simulink model "model3"  (R2024b)
settings: Solver=VariableStepAuto  StartTime=0.0  StopTime=10  RelTol=1e-3
values from neighbouring files (symbols this model uses):
  A = [-3, 2; 1, -2]    [domaci3.m]
  B = [0; 2]    [domaci3.m]
  C = [0, 1]    [domaci3.m]
  K = acker(A, B, p_cl)    [domaci3.m]
  kr = 1 / dcgain(s * G0 / s)    [domaci3.m]
  L = acker(A', C', p_est)'    [domaci3.m]
  R = 5    [domaci3.m]
settings Model: Creator=neso  LastModifiedBy=neso

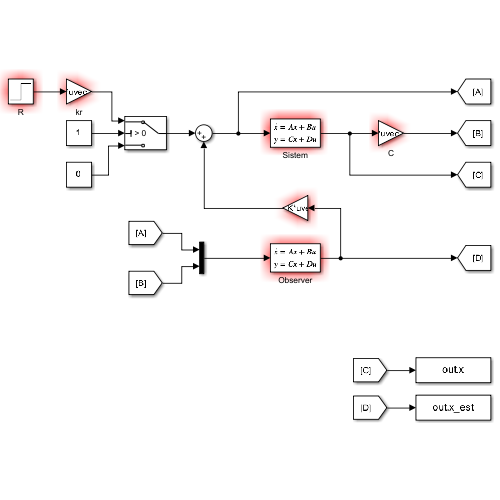
[thumbnail: Simulink's stored preview of the top-level diagram]
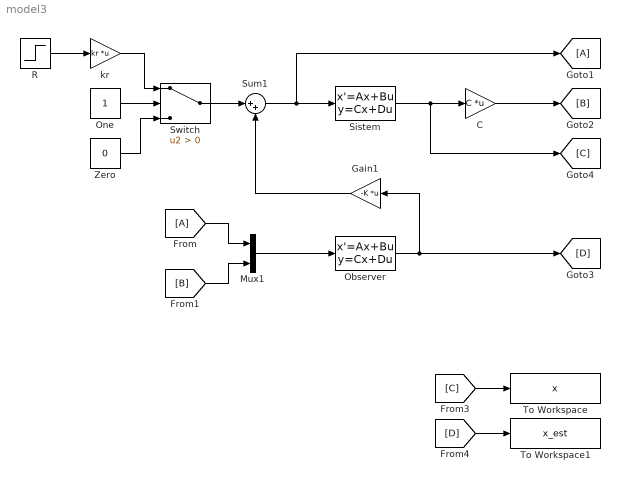
== system model3 ==
  C : Gain  Gain=C  Multiplication=Matrix(K*u) (u vector)
  From : From
  Gain1 : Gain  Gain=-K  Multiplication=Matrix(K*u) (u vector)
  Goto1 : Goto
  Mux1 : Mux  Inputs=2
  Observer : StateSpace  A=A - L .* C  B=[B, L]  C=[1, 0; 0, 1]  D=[0, 0; 0, 0]  InitialCondition=[0; 0]
  One : Constant  OutDataTypeStr=Inherit: Inherit via back propagation
  R : Step  Time=0  After=R  SampleTime=0
  Sistem : StateSpace  A=A  B=B  C=[1, 0; 0, 1]  D=[0; 0]  InitialCondition=[2; -2]
  Sum1 : Sum  Inputs=|++
  Switch : Switch  Criteria=u2 > Threshold  SaturateOnIntegerOverflow=off  InputSameDT=off
  To Workspace : ToWorkspace  VariableName=x  SaveFormat=Timeseries  SampleTime=-1
  To Workspace1 : ToWorkspace  VariableName=x_est  SaveFormat=Timeseries  SampleTime=-1
  Zero : Constant  Value=0  OutDataTypeStr=Inherit: Inherit via back propagation
  kr : Gain  Gain=kr  Multiplication=Matrix(K*u) (u vector)
  wires:
  R/1 -> kr/1
  Sum1/1 -> Goto1/1, Sistem/1
  Gain1/1 -> Sum1/2
  Observer/1 -> [D], Gain1/1
  Mux1/1 -> Observer/1
  From/1 -> Mux1/1
  [B] -> Mux1/2
  Switch/1 -> Sum1/1
  kr/1 -> Switch/1
  One/1 -> Switch/2
  Zero/1 -> Switch/3
  [C] -> To Workspace/1
  [D] -> To Workspace1/1
  Sistem/1 -> [C], C/1
  C/1 -> [B]
